simulink model "SimulacionPV"  (R2022a)
settings: Solver=VariableStepAuto  StartTime=0.0  StopTime=30  RelTol=1e-3
libraries: simulink x1
settings Model: Creator=Joaco  LastModifiedBy=Joaco

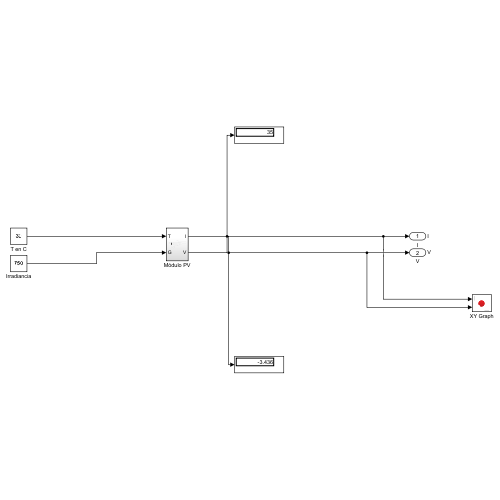
[thumbnail: Simulink's stored preview of the top-level diagram]
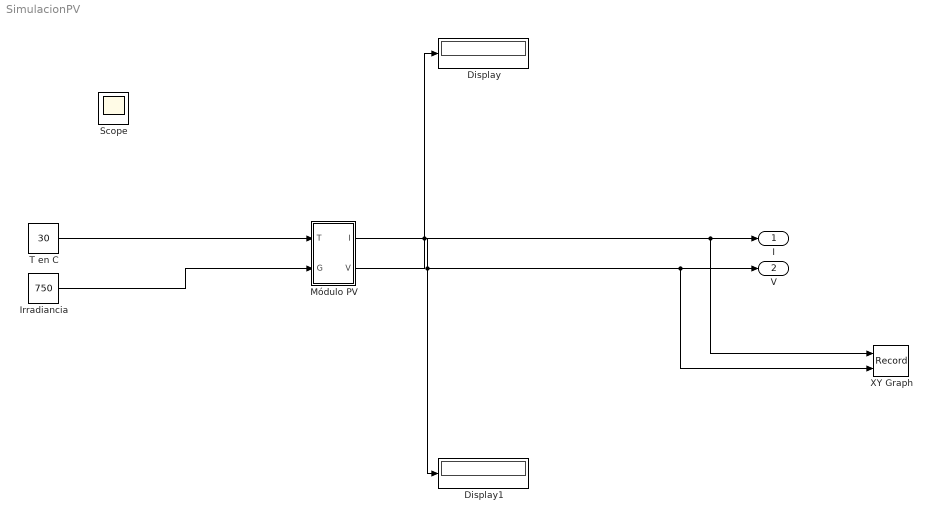
== system SimulacionPV ==
  Display : Display
  Display1 : Display
  Irradiancia : Constant  Value=750
  Módulo PV : Subsystem
  T en C : Constant  Value=30
  XY Graph : Record  FileSettingsInternal="{\"entries\":[{\"content\":{\"excelSettings\":{\"content\":{},\"type\":\"Streamout.ExcelSettings\"}},\"type\":\"Streamout.FileSettingStorage\",\"uuid\":\"78944f17-0da0-4f50-996c-895c94181894\"}],\"packageUris\":[\"http://schema.mathworks.com/mf0/streamout_blocks/R2020a\"],\"version\":\"1.0\"}"  Layout=[1 1]  SignalsInternal="{\"entries\":[{\"content\":{\"signals\":[{\"content\":{\"blockPath\":[\"SimulacionPV/XY Graph\"],\"channel\":[],\"dimensions\":[1],\"domain\":\"SimulacionPV/XY Graph\",\"lineColor\":\"#a2142f\",\"plots\":[1],\"port\":1,\"sid\":[\"\"],\"signalID\":2049,\"signalName\":\"Módulo PV:2\"},\"type\":\"RecordBlkView.Signal\",\"uuid\":\"392e2603-8fc2-47e8-942a-ec50105226ba\"},{\"content\":{\"blockPath\":[\"SimulacionPV/XY Graph\"],\"channel\":[],\"dimensions\":[1],\"domain\":\"SimulacionPV/XY Graph\",\"lineColor\":\"#139fff\",\"plots\":[1],\"port\":2,\"sid\":[\"\"],\"signalID\":2053,\"signalName\":\"Módulo PV:1\"},\"type\":\"RecordBlkView.Signal\",\"uuid\":\"ba175721-0089-4780-be35-61e3ccb90ab9\"}]},\"type\":\"RecordBlkView.InputSignals\",\"uuid\":\"a7c09eeb-a234-4d7f-adcc-d392da18d90e\"}],\"packageUris\":[\"http://schema.mathworks.com/mf0/streamout_blocks/R2020a\"],\"version\":\"1.0\"}"  VisualizationBindings="{\"xyplotplugin\":{\"info\":[{\"series\":[{\"bindingParametersList\":[{\"parameter\":\"X-Axis\",\"signalID\":2049,\"signalName\":\"Módulo PV:2\"},{\"parameter\":\"Y-Axis\",\"signalID\":2053,\"signalName\":\"Módulo PV:1\"}],\"seriesID\":403}],\"subplotID\":1}]}}"  CompatibilityTag=XY
  I : Outport  SignalName=I
  V : Outport  Port=2  SignalName=V
  Scope : Scope
  wires:
  Módulo PV/2(V) -> Display/1, XY Graph/1, I/1
  Módulo PV/1(I) -> Display1/1, XY Graph/2, V/1
  T en C/1 -> Módulo PV/1(T)
  Irradiancia/1 -> Módulo PV/2(G)

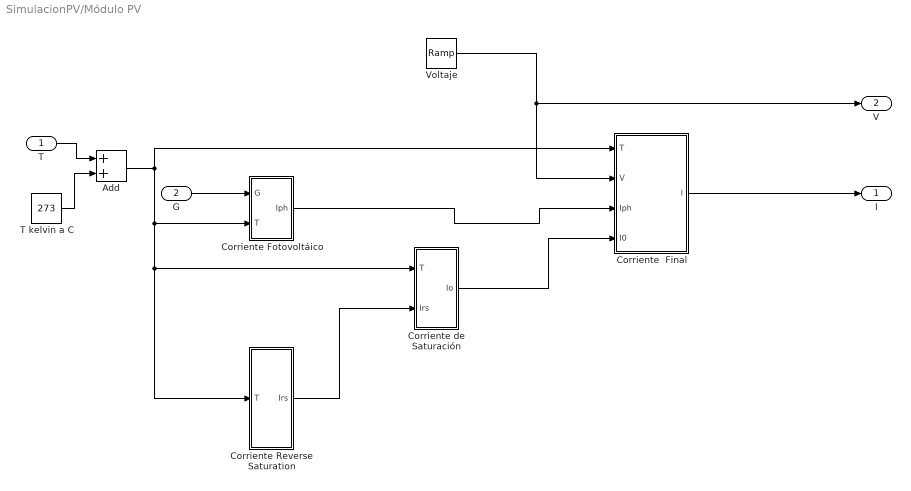
== system SimulacionPV/Módulo PV ==
  T : Inport
  G : Inport  Port=2
  Add : Sum
  Corriente  Final : Subsystem
  Corriente Fotovoltáico : Subsystem
  Corriente Reverse Saturation : Subsystem
  Corriente de Saturación : Subsystem
  T kelvin a C : Constant  Value=273
  Voltaje : simulink/Sources/Ramp  slope=1  start=0  InitialOutput=1
  I : Outport
  V : Outport  Port=2
  wires:
  Add/1 -> Corriente Fotovoltáico/2(T), Corriente de Saturación/1(T), Corriente Reverse Saturation/1(T), Corriente  Final/1(T)
  Corriente Fotovoltáico/1(Iph) -> Corriente  Final/3(Iph)
  Voltaje/1 -> V/1, Corriente  Final/2(V)
  Corriente de Saturación/1(Io) -> Corriente  Final/4(I0)
  Corriente  Final/1(I) -> I/1
  T kelvin a C/1 -> Add/2
  Corriente Reverse Saturation/1(Irs) -> Corriente de Saturación/2(Irs)
  T/1 -> Add/1
  G/1 -> Corriente Fotovoltáico/1(G)

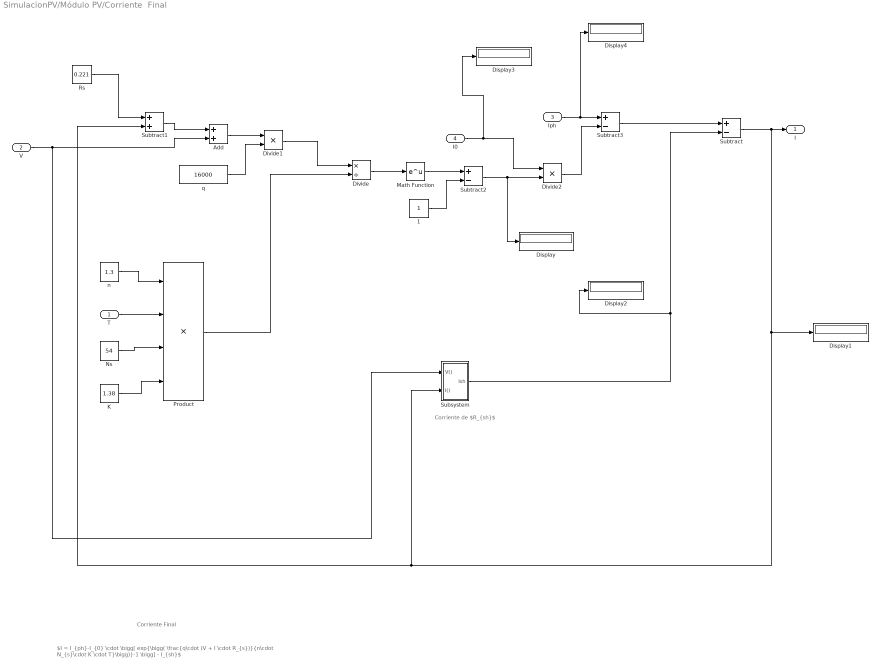
== system SimulacionPV/Módulo PV/Corriente  Final ==
  note: $I = I_{ph}-I_{0} \cdot \bigg[ exp{\bigg( \frac{q\cdot (V + I \cdot R_{s})}{n\cdot N_{s}\cdot K \cdot T}\bigg)}-1 \bigg] - I_{sh}$
  note: Corriente de $R_{sh}$
  note: Corriente Final
  T : Inport
  V : Inport  Port=2
  Iph : Inport  Port=3
  I0 : Inport  Port=4
  1 : Constant
  Add : Sum
  Display{,1..4} (5 alike) : Display
  Divide : Product  Inputs=*/
  Divide1 : Product  Inputs=**
  Divide2 : Product  Inputs=**
  K : Constant  Value=1.38
  Math Function : Math
  Ns : Constant  Value=54
  Product : Product  Inputs=4
  Rs : Constant  Value=0.221
  Subsystem : Subsystem
  Subtract : Sum  Inputs=+-
  Subtract1 : Sum
  Subtract2 : Sum  Inputs=+-
  Subtract3 : Sum  Inputs=+-
  n : Constant  Value=1.3
  q : Constant  Value=16000
  I : Outport
  wires:
  Rs/1 -> Subtract1/1
  Subtract/1 -> Display1/1, Subsystem/2(I()), Subtract1/2, I/1
  Subtract1/1 -> Add/1
  n/1 -> Product/1
  T/1 -> Product/2
  Ns/1 -> Product/3
  K/1 -> Product/4
  Product/1 -> Divide/2
  Divide/1 -> Math Function/1
  Math Function/1 -> Subtract2/1
  1/1 -> Subtract2/2
  Add/1 -> Divide1/1
  q/1 -> Divide1/2
  Divide1/1 -> Divide/1
  I0/1 -> Display3/1, Divide2/1
  Subtract2/1 -> Display/1, Divide2/2
  V/1 -> Subsystem/1(V()), Add/2
  Iph/1 -> Display4/1, Subtract3/1
  Divide2/1 -> Subtract3/2
  Subtract3/1 -> Subtract/1
  Subsystem/1(Ish) -> Subtract/2, Display2/1

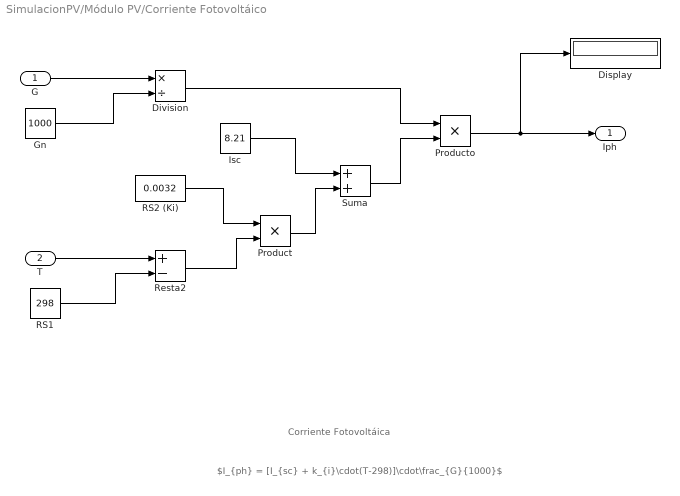
== system SimulacionPV/Módulo PV/Corriente Fotovoltáico ==
  note: Corriente Fotovoltáica
  note: $I_{ph} = [I_{sc} + k_{i}\cdot(T-298)]\cdot\frac_{G}{1000}$
  G : Inport
  T : Inport  Port=2
  Display : Display
  Division : Product  Inputs=*/
  Gn : Constant  Value=1000
  Isc : Constant  Value=8.21
  Product : Product
  Producto : Product
  RS1 : Constant  Value=298
  RS2 (Ki) : Constant  Value=0.0032
  Resta2 : Sum  Inputs=+-
  Suma : Sum
  Iph : Outport
  wires:
  Product/1 -> Suma/2
  Producto/1 -> Iph/1, Display/1
  RS2 (Ki)/1 -> Product/1
  Gn/1 -> Division/2
  RS1/1 -> Resta2/2
  Division/1 -> Producto/1
  G/1 -> Division/1
  Suma/1 -> Producto/2
  Isc/1 -> Suma/1
  Resta2/1 -> Product/2
  T/1 -> Resta2/1

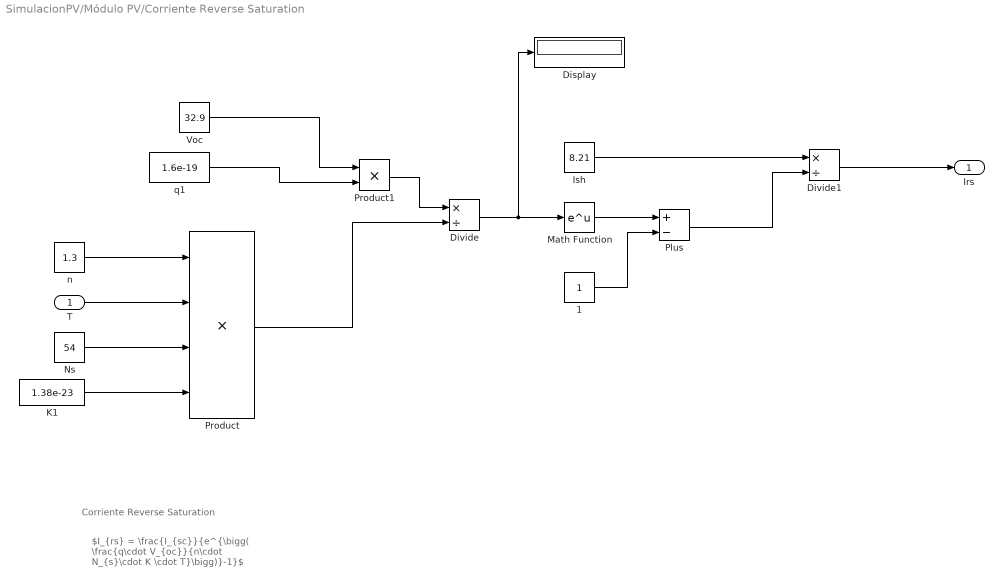
== system SimulacionPV/Módulo PV/Corriente Reverse Saturation ==
  note: Corriente Reverse Saturation
  note: $I_{rs} = \frac{I_{sc}}{e^{\bigg( \frac{q\cdot V_{oc}}{n\cdot N_{s}\cdot K \cdot T}\bigg)}-1}$
  T : Inport
  1 : Constant
  Display : Display
  Divide : Product  Inputs=*/
  Divide1 : Product  Inputs=*/
  Ish : Constant  Value=8.21
  K1 : Constant  Value=1.38e-23
  Math Function : Math
  Ns : Constant  Value=54
  Plus : Sum  Inputs=+-
  Product : Product  Inputs=4
  Product1 : Product
  Voc : Constant  Value=32.9
  n : Constant  Value=1.3
  q1 : Constant  Value=1.6e-19
  Irs : Outport
  wires:
  n/1 -> Product/1
  T/1 -> Product/2
  Ns/1 -> Product/3
  K1/1 -> Product/4
  Product/1 -> Divide/2
  q1/1 -> Product1/2
  Voc/1 -> Product1/1
  Product1/1 -> Divide/1
  Divide/1 -> Display/1, Math Function/1
  Math Function/1 -> Plus/1
  1/1 -> Plus/2
  Plus/1 -> Divide1/2
  Ish/1 -> Divide1/1
  Divide1/1 -> Irs/1

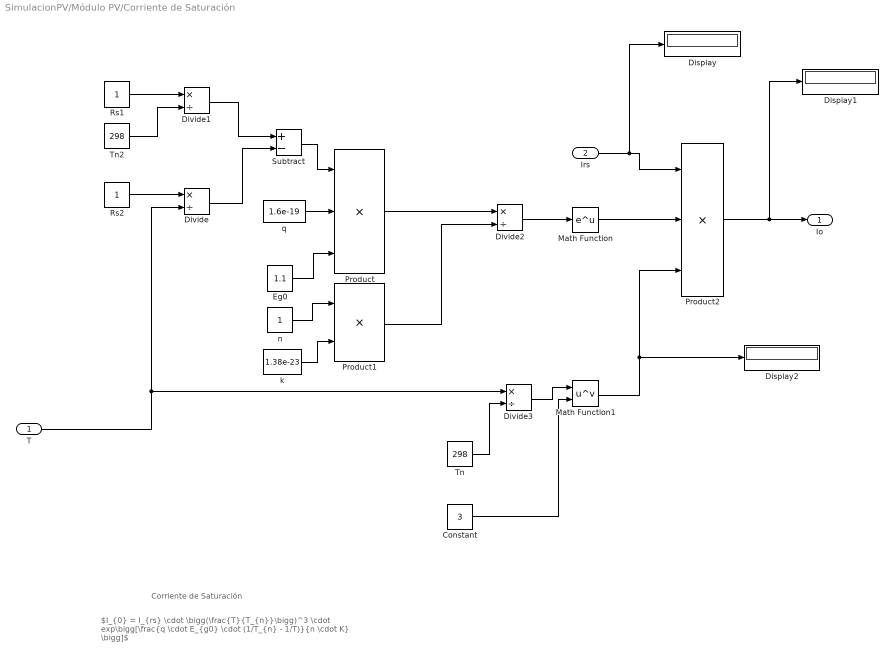
== system SimulacionPV/Módulo PV/Corriente de Saturación ==
  note: Corriente de Saturación
  note: $I_{0} = I_{rs} \cdot \bigg(\frac{T}{T_{n}}\bigg)^3 \cdot exp\bigg[\frac{q \cdot E_{g0} \cdot (1/T_{n} - 1/T)}{n \cdot K} \bigg]$
  T : Inport
  Irs : Inport  Port=2
  Constant : Constant  Value=3
  Display : Display
  Display1 : Display
  Display2 : Display
  Divide{,1..3} (4 alike) : Product  Inputs=*/
  Eg0 : Constant  Value=1.1
  Math Function : Math
  Math Function1 : Math  Operator=pow
  Product : Product  Inputs=3
  Product1 : Product
  Product2 : Product  Inputs=3
  Rs1 : Constant
  Rs2 : Constant
  Subtract : Sum  Inputs=+-
  Tn : Constant  Value=298
  Tn2 : Constant  Value=298
  k : Constant  Value=1.38e-23
  n : Constant
  q : Constant  Value=1.6e-19
  Io : Outport
  wires:
  T/1 -> Divide3/1, Divide/2
  Rs2/1 -> Divide/1
  Divide1/1 -> Subtract/1
  Divide/1 -> Subtract/2
  Subtract/1 -> Product/1
  q/1 -> Product/2
  Eg0/1 -> Product/3
  Product/1 -> Divide2/1
  n/1 -> Product1/1
  k/1 -> Product1/2
  Product1/1 -> Divide2/2
  Divide2/1 -> Math Function/1
  Tn/1 -> Divide3/2
  Divide3/1 -> Math Function1/1
  Constant/1 -> Math Function1/2
  Irs/1 -> Display/1, Product2/1
  Math Function/1 -> Product2/2
  Math Function1/1 -> Display2/1, Product2/3
  Product2/1 -> Display1/1, Io/1
  Rs1/1 -> Divide1/1
  Tn2/1 -> Divide1/2

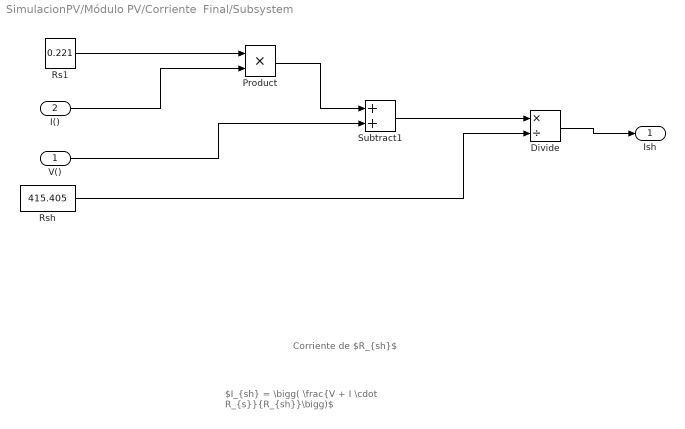
== system SimulacionPV/Módulo PV/Corriente  Final/Subsystem ==
  note: $I_{sh} = \bigg( \frac{V + I \cdot R_{s}}{R_{sh}}\bigg)$
  note: Corriente de $R_{sh}$
  V() : Inport
  I() : Inport  Port=2
  Divide : Product  Inputs=*/
  Product : Product
  Rs1 : Constant  Value=0.221
  Rsh : Constant  Value=415.405
  Subtract1 : Sum
  Ish : Outport
  wires:
  V()/1 -> Subtract1/2
  Rsh/1 -> Divide/2
  Divide/1 -> Ish/1
  Product/1 -> Subtract1/1
  Rs1/1 -> Product/1
  Subtract1/1 -> Divide/1
  I()/1 -> Product/2
